simulink model "Modulator_Xilinx_Verilog"  (Simulink 7.8)
settings: Solver=VariableStepDiscrete  StartTime=0.0  StopTime=100/25000000  RelTol=1e-3
undefined symbols (not defined in the file): gcbh, xlBlockLoadCallback, xlipgetpartsetting
libraries: xbsIndex_r4 x11
settings Model: Creator=Cedric  LastModifiedBy=Cedric

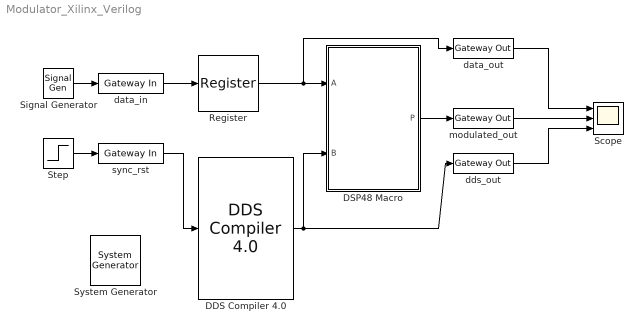
== system Modulator_Xilinx_Verilog ==
  " System Generator" : xbsIndex_r4/ System Generator  Tag=genX  xilinxfamily=virtex6  part=xc6vlx240t  speed=-1  package=ff1156  synthesis_tool=XST  clock_wrapper=Clock Enables  directory=./netlist  proj_type=Project Navigator  Synth_file=XST Defaults  Impl_file=ISE Defaults  testbench=off  simulink_period=1/25000000  sysclk_period=10  dcm_input_clock_period=10  incr_netlist=off  trim_vbits=Everywhere in SubSystem  dbl_ovrd=According to Block Masks  core_generation=According to Block Masks  run_coregen=off  deprecated_control=off  eval_field=0  block_type=sysgen
  "DDS Compiler 4.0 " : xbsIndex_r4/DDS Compiler 4.0   partspresent=Phase_Generator_and_SIN_COS_LUT  dds_clock_rate=100  channels=1  parameter_entry=System_Parameters  spurious_free_dynamic_range=36  frequency_resolution=0.4  noise_shaping=None  phase_width=28  output_width=6  output_selection=Sine  negative_sine=off  negative_cosine=off  amplitude_mode=Full_Range  memory_type=Block_ROM  optimization_goal=Auto  dsp48_use=Maximal  latency_configuration=Auto  latency=2  has_phase_out=off  sclr_pin=on  clock_enable=off  rfd=off  rdy=off  channel_pin=off  explicit_period=off  period=1  phase_increment=Fixed  output_frequency1=5  output_frequency2=0  output_frequency3=0  output_frequency4=0  output_frequency5=0  output_frequency6=0  output_frequency7=0  output_frequency8=0  output_frequency9=0  output_frequency10=0  output_frequency11=0  output_frequency12=0  output_frequency13=0  output_frequency14=0  output_frequency15=0  output_frequency16=0  pinc1='0'  pinc2='0'  pinc3='0'  pinc4='0'  pinc5='0'  pinc6='0'  pinc7='0'  pinc8='0'  pinc9='0'  pinc10='0'  pinc11='0'  pinc12='0'  pinc13='0'  pinc14='0'  pinc15='0'  pinc16='0'  phase_offset=None  phase_offset_angles1=0  phase_offset_angles2=0  phase_offset_angles3=0  phase_offset_angles4=0  phase_offset_angles5=0  phase_offset_angles6=0  phase_offset_angles7=0  phase_offset_angles8=0  phase_offset_angles9=0  phase_offset_angles10=0  phase_offset_angles11=0  phase_offset_angles12=0  phase_offset_angles13=0  phase_offset_angles14=0  phase_offset_angles15=0  phase_offset_angles16=0  poff1='0'  poff2='0'  poff3='0'  poff4='0'  poff5='0'  poff6='0'  poff7='0'  poff8='0'  poff9='0'  poff10='0'  poff11='0'  poff12='0'  poff13='0'  poff14='0'  poff15='0'  poff16='0'  por_mode=false  gui_behaviour=Sysgen  ip_name=DDS Compiler  ip_version=4.0  dsptool_ready=true  wrapper_available=true  port_translation_map={ 'ce' => 'en', 'sclr' => 'rst' }  ipcore_xco_need_fpga_part=true  ipcore_fpga_part=xlipgetpartsetting(gcb, {'virtex4', 'xc4vsx35', '-10', 'ff668'})  ipcore_usecache=true  ipcore_useipmodelcache=true  ipcore_verbose=false  block_type=dds_compiler_v4_0
  DSP48 Macro : Subsystem  LoadFcn=xlBlockLoadCallback(gcbh);  mask(Xilinx DSP48 Macro Block){infoedit=Macro function to simplify use of the DSP48 primitive, especially as a dynamic operator, portalist=A, portblist=B, portclist=No, instrlist=|, pipeline_sgadvanced=, pipeline=Custom, pipeachoices_sgadvanced=, pipeachoices=1, pipebchoices_sgadvanced=, pipebchoices=1, pipecchoices_sgadvanced=, pipecchoices=on, pipepchoices_sgadvanced=, pipepchoices=on, pipemchoices_sgadvanced=, pipemchoices=on, pipectrlchoices_sgadvanced=, pipectrlchoices=on, pipemuxachoices_sgadvanced=, pipemuxachoices=0, pipemuxbchoices_sgadvanced=, pipemuxbchoices=0, pipemuxcchoices_sgadvanced=, pipemuxcchoices=0, pipemuxctrlchoices_sgadvanced=, pipemuxctrlchoices=0, pipeline_array_flag_sgadvanced=, pipeline_array_flag=off, custom_pipeline_cache=[1  1  1  1  1  1  0  0  0  0], precision_sgadvanced=, precision=Full, arith_type_sgadvanced=, arith_type=Unsigned, n_bits=8, bin_pt=2, bcout_sgadvanced=, bcout=off, acout_sgadvanced=, acout=off, carryout_sgadvanced=, carryout=off, carrycascout_sgadvanced=, carrycascout=off, pcout_sgadvanced=, pcout=off, rst_all_sgadvanced=, rst_all=off, rst_a_sgadvanced=, rst_a=off, rst_b_sgadvanced=, rst_b=off, rst_c_sgadvanced=, rst_c=off, rst_m_sgadvanced=, rst_m=off, rst_p_sgadvanced=, rst_p=off, rst_ctrl_sgadvanced=, rst_ctrl=off, ce_all_sgadvanced=, ce_all=off, ce_a_sgadvanced=, ce_a=off, ce_b_sgadvanced=, ce_b=off, ce_c_sgadvanced=, ce_c=off, ce_m_sgadvanced=, ce_m=off, ce_p_sgadvanced=, ce_p=off, ce_ctrl_sgadvanced=, ce_ctrl=off, dbl_ovrd_sgadvanced=, dbl_ovrd=off, synth_opt_sgadvanced=, synth_opt=on, errorlist=false, statestr=8748f9e4e14b4b54c46918fee19c673c, explicit_period=, period=1, maskdoc=, has_advanced_control=0, sggui_pos=-1,-1,-1,-1, block_type=dsp48macro, block_version=8.2.1, sg_icon_stat=90,142,2,1,white,blue,0,7afd0e130bd830a51d6376b21eaeb333,right,,[ ],[ ], sg_mask_display=|, sg_list_contents=, sg_blockgui_xml=}
      mask instrlist=|
      | <!DOCTYPE HTML PUBLIC "-//W3C//DTD HTML 4.0//EN" "http://www.w3.org/TR/REC-html40/strict.dtd">
      | <html><head><meta name="qrichtext" content="1" /><style type="text/css">
      | p, li { white-space: pre-wrap; }
      | </style></head><body style=" font-family:'MS Shell Dlg 2'; font-size:8.25pt; font-weight:400; font-style:normal;">
      | <p style=" margin-top:12px; margin-bottom:12px; margin-left:0px; margin-right:0px; -qt-block-indent:0; text-indent:0px;"><span style=" font-family:'MS Shell Dlg'; font-size:8pt;">P=A*B</span></p></body></html>
      mask sg_mask_display=|
      | fprintf('','COMMENT: begin icon graphics');
      | patch([0 90 90 0 0 ],[0 0 142 142 0 ],[0.77 0.82 0.91 ]);
      | plot([0 90 90 0 0 ],[0 0 142 142 0 ]);
      | patch([18.3 35.64 47.64 59.64 71.64 47.64 30.3 18.3 ],[84.32 84.32 96.32 84.32 96.32 96.32 96.32 84.32 ],[1 1 1 ]);
      | patch([30.3 47.64 35.64 18.3 30.3 ],[72.32 72.32 84.32 84.32 72.32 ],[0.931 0.946 0.973 ]);
      | patch([18.3 35.64 47.64 30.3 18.3 ],[60.32 60.32 72.32 72.32 60.32 ],[1 1 1 ]);
      | patch([30.3 71.64 59.64 47.64 35.64 18.3 30.3 ],[48.32 48.32 60.32 48.32 60.32 60.32 48.32 ],[0.931 0.946 0.973 ]);
      | fprintf('','COMMENT: end icon graphics');
      | fprintf('','COMMENT: begin icon text');
      | color('black');port_label('input',1,'A');
      | color('black');port_label('input',2,'B');
      | color('black');port_label('output',1,'P');
      | fprintf('','COMMENT: end icon text');
      mask prompts: infoedit ""; portalist "Inputs to port <tt>A</tt>"; portblist "Inputs to port <tt>B</tt>"; portclist "Inputs to port <tt>C</tt>"; instrlist "Instructions"; pipeline_sgadvanced ""; pipeline "Pipeline options"; pipeachoices_sgadvanced ""; pipeachoices "<tt>A</tt>"; pipebchoices_sgadvanced ""; pipebchoices "<tt>B</tt>"; pipecchoices_sgadvanced ""; pipecchoices "<tt>C</tt>"; pipepchoices_sgadvanced ""; pipepchoices "<tt>P</tt>"; pipemchoices_sgadvanced ""; pipemchoices "Multiplier"; pipectrlchoices_sgadvanced ""; pipectrlchoices "Controls (<tt>opmode</tt>, <tt>subtract</tt>,<br> <tt>carry_in</tt>, <tt>carry_in_sel</tt>)"; pipemuxachoices_sgadvanced ""; pipemuxachoices "MuxA"; pipemuxbchoices_sgadvanced ""; pipemuxbchoices "MuxB"; pipemuxcchoices_sgadvanced ""; pipemuxcchoices "MuxC"; pipemuxctrlchoices_sgadvanced ""; pipemuxctrlchoices "MuxCtrl"; pipeline_array_flag_sgadvanced ""; pipeline_array_flag "Define Using Array"; custom_pipeline_cache "Custom Pipeline Options([A,B,C,P,Ctrl,M,MuxA,MuxB,MuxC,MuxCtrl])"; precision_sgadvanced ""; arith_type_sgadvanced ""; arith_type "Output type"; n_bits "Number of bits"; bin_pt "Binary point"; bcout_sgadvanced ""; bcout "<tt>BCOUT</tt>"; acout_sgadvanced ""; acout "<tt>ACOUT</tt>"; carryout_sgadvanced ""; carryout "<tt>CARRYOUT</tt>"; carrycascout_sgadvanced ""; carrycascout "<tt>CARRYCASCOUT</tt>"; pcout_sgadvanced ""; pcout "<tt>PCOUT</tt>"; rst_all_sgadvanced ""; rst_all "<tt>Global Reset</tt>"; rst_a_sgadvanced ""; rst_a "Reset port for <tt>A</tt>"; rst_b_sgadvanced ""; rst_b "Reset port for <tt>B</tt>"; rst_c_sgadvanced ""; rst_c "Reset port for <tt>C</tt>"; rst_m_sgadvanced ""; rst_m "Reset port for multiplier"; rst_p_sgadvanced ""; rst_p "Reset port for <tt>P</tt>"; rst_ctrl_sgadvanced ""; rst_ctrl "Reset port for controls <br> (<tt>opmode</tt>, <tt>subtract</tt>,<br> <tt>carry_in</tt>, <tt>carry_in_sel</tt>)"; ce_all_sgadvanced ""; ce_all "<tt>Global Enable</tt>"; ce_a_sgadvanced ""; ce_a "Enable port for <tt>A</tt>"; ce_b_sgadvanced ""; ce_b "Enable port for <tt>B</tt>"; ce_c_sgadvanced ""; ce_c "Enable port for <tt>C</tt>"; ce_m_sgadvanced ""; ce_m "Enable port for multiplier"; ce_p_sgadvanced ""; ce_p "Enable port for <tt>P</tt>"; ce_ctrl_sgadvanced ""; ce_ctrl "Enable port for controls <br> (<tt>opmode</tt>, <tt>subtract</tt>,<br> <tt>carry_in</tt>, <tt>carry_in_sel</tt>)"; dbl_ovrd_sgadvanced ""; dbl_ovrd "Override with doubles"; synth_opt_sgadvanced ""; synth_opt "Use DSP48"; errorlist ""; statestr ""; explicit_period ""; period ""; maskdoc ""; has_advanced_control ""; sggui_pos ""; block_type ""; block_version ""; sg_icon_stat ""; sg_mask_display ""; sg_list_contents ""; sg_blockgui_xml ""
      mask help: Macro function to simplify use of the DSP48 primitive, especially as a dynamic operator
      mask init:
      | try
      |   tmp_gcb = gcb;
      |   tmp_gcbh = gcbh;
      |   if (strcmp('SysGenIndex',get_param(bdroot(tmp_gcbh),'tag')) && ~isempty(regexp(bdroot(tmp_gcb), '^xbs', 'once')))
      |     return;
      |   end;
      |   xlMungeMaskParams;
      | 
      |   block_type='dsp48macro';
      | 
      |   serialized_declarations = '{''block_type''=>''String''}';
      |   xldsp48macro_init();
      |   ptable_ = xlblockprep(get_param(tmp_gcb, 'MaskWSVariables'));
      |   try
      |     xlBlockMoveCallback(tmp_gcbh);
      |   catch 
      |      clear global xl_updateicon_recursion_guard;
      |   end;
      | catch
      |   global dbgsysgen;
      |   if(~isempty(dbgsysgen) && dbgsysgen)
      |     e = regexprep(lasterr, '\n', '\nError: ');
      |     disp(['Error: While running MaskInit code on block ' tmp_gcb ': ' e]);
      |     error(e);
      |   end
      | end
      settings: CopyFcn=tmp_gcbh = gcbh;set_param(tmp_gcbh,'linkstatus','none');xlBlockMoveCallback(gcbh);  DeleteFcn=xlDestroyGui(gcbh);  ModelCloseFcn=xlDestroyGui(gcbh);  PreSaveFcn=xlBlockPreSaveCallback(gcbh);  PostSaveFcn=xlBlockPostSaveCallback(gcbh);  DestroyFcn=xlDestroyGui(gcbh);  OpenFcn=xlOpenGui(gcbh, 'dsp48macro_gui.xml', @dsp48macroenablement, @dsp48macroaction)  CloseFcn=xlDestroyGui(gcbh);  MoveFcn=xlBlockMoveCallback(gcbh);
      mask Help: eval('');xlDoc('-book','sysgen','-topic','DSP48_Macro');
      mask StyleString: edit,edit,edit,edit,edit,edit,popup(External Registers|No External Registers|Custom),edit,popup(0|1|2),edit,popup(0|1|2),edit,checkbox,edit,checkbox,edit,checkbox,edit,checkbox,edit,popup(0|1|2),edit,popup(0|1|2),edit,popup(0|1|2),edit,popup(0|1|2),edit,checkbox,edit,edit,popup(Full|User Defined),edit,popup(Signed  (2's comp)|Unsigned),edit,edit,edit,checkbox,edit,checkbox,edit,checkbox,edit,checkbox,edit,checkbox,edit,checkbox,edit,checkbox,edit,checkbox,edit,checkbox,edit,checkbox,edit,checkbox,edit,checkbox,edit,checkbox,edit,checkbox,edit,checkbox,edit,checkbox,edit,checkbox,edit,checkbox,edit,checkbox,edit,checkbox,edit,checkbox,edit,edit,edit,edit,edit,edit,edit,edit,edit,edit,edit,edit,edit
      mask Display:
      | fprintf('','COMMENT: begin icon graphics');
      | patch([0 90 90 0 0 ],[0 0 142 142 0 ],[0.77 0.82 0.91 ]);
      | plot([0 90 90 0 0 ],[0 0 142 142 0 ]);
      | patch([18.3 35.64 47.64 59.64 71.64 47.64 30.3 18.3 ],[84.32 84.32 96.32 84.32 96.32 96.32 96.32 84.32 ],[1 1 1 ]);
      | patch([30.3 47.64 35.64 18.3 30.3 ],[72.32 72.32 84.32 84.32 72.32 ],[0.931 0.946 0.973 ]);
      | patch([18.3 35.64 47.64 30.3 18.3 ],[60.32 60.32 72.32 72.32 60.32 ],[1 1 1 ]);
      | patch([30.3 71.64 59.64 47.64 35.64 18.3 30.3 ],[48.32 48.32 60.32 48.32 60.32 60.32 48.32 ],[0.931 0.946 0.973 ]);
      | fprintf('','COMMENT: end icon graphics');
      | fprintf('','COMMENT: begin icon text');
      | color('black');port_label('input',1,'A');
      | color('black');port_label('input',2,'B');
      | color('black');port_label('output',1,'P');
      | fprintf('','COMMENT: end icon text');
  Register : xbsIndex_r4/Register  init=0  rst=off  en=off  dbl_ovrd=off  block_type=register
  Scope : Scope  NumInputPorts=3
      settings: YMin=-5~-5~-5  YMax=5~5~5
  Signal Generator : SignalGenerator  WaveForm=square  Frequency=500000
  Step : Step  Time=1/25000000  Before=1  After=0  SampleTime=1/25000000
  data_in : xbsIndex_r4/Gateway In  gui_display_data_type=Fixed-point  arith_type="Signed  (2's comp)"  n_bits=16  bin_pt=14  preci_type=Single  exp_width=8  frac_width=24  quantization="Round  (unbiased: +/- Inf)"  overflow=Saturate  period=1/25000000  dbl_ovrd=off  timing_constraint=None  locs_specified=off  LOCs={}  UseAsADC=off  ADCChannel='1'  inherit_from_input=off  hdl_port=on  block_type=gatewayin
  data_out : xbsIndex_r4/Gateway Out  inherit_from_input=off  hdl_port=on  timing_constraint=None  locs_specified=off  LOCs={}  UseAsDAC=off  DACChannel='1'  block_type=gatewayout
  dds_out : xbsIndex_r4/Gateway Out  inherit_from_input=off  hdl_port=on  timing_constraint=None  locs_specified=off  LOCs={}  UseAsDAC=off  DACChannel='1'  block_type=gatewayout
  modulated_out : xbsIndex_r4/Gateway Out  inherit_from_input=off  hdl_port=on  timing_constraint=None  locs_specified=off  LOCs={}  UseAsDAC=off  DACChannel='1'  block_type=gatewayout
  sync_rst : xbsIndex_r4/Gateway In  gui_display_data_type=Boolean  arith_type=Boolean  n_bits=16  bin_pt=14  preci_type=Single  exp_width=8  frac_width=24  quantization="Round  (unbiased: +/- Inf)"  overflow=Saturate  period=1/25000000  dbl_ovrd=off  timing_constraint=None  locs_specified=off  LOCs={}  UseAsADC=off  ADCChannel='1'  inherit_from_input=off  hdl_port=on  block_type=gatewayin
  wires:
  data_in/1 -> Register/1
  Signal Generator/1 -> data_in/1
  Register/1 -> DSP48 Macro/1(A), data_out/1
  data_out/1 -> Scope/1
  DSP48 Macro/1(P) -> modulated_out/1
  modulated_out/1 -> Scope/2
  dds_out/1 -> Scope/3
  sync_rst/1 -> "DDS Compiler 4.0 "/1
  "DDS Compiler 4.0 "/1 -> DSP48 Macro/2(B), dds_out/1
  Step/1 -> sync_rst/1

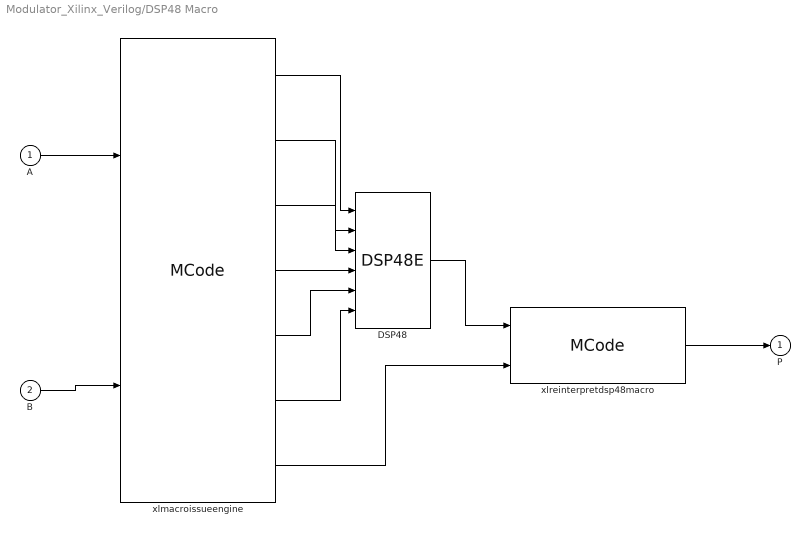
== system Modulator_Xilinx_Verilog/DSP48 Macro ==
  A : Inport
  B : Inport  Port=2
  DSP48 : xbsIndex_r4/DSP48E  use_a=Direct from A Port  use_b=Direct from B Port  reset_preg=off  pattern_from_creg=on  pattern='000000000000'  mask_from_creg=on  pattern_mask='000000000000'  sel_rounding_mask=Select mask  use_op=off  use_creg=off  rst_all=off  en_all=off  use_pcin=off  use_carrycascin=off  use_multsignin=off  use_carryout=off  use_patterndetect=off  use_patternbdetect=off  use_overflow=off  use_underflow=off  use_acout=off  use_bcout=off  use_pcout=off  use_multsignout=off  use_carrycascout=off  pipeline_a=1  pipeline_b=1  pipeline_acout=1  pipeline_bcout=1  pipeline_c=off  pipeline_p=on  pipeline_mult=on  pipeline_opmode=on  pipeline_alumode=on  pipeline_carryin=on  pipeline_carryinsel=on  rst_a=off  rst_b=off  rst_c=off  rst_mult=off  rst_p=off  rst_carry_in=off  rst_alumode=off  rst_ctrl=off  en_a1=off  en_a2=off  en_b1=off  en_b2=off  en_c=off  en_mult=off  en_p=off  en_carry_in=off  en_alumode=off  en_multcarryin=off  en_ctrl=off  use_synth_model=off  addsub_mode=ONE48  xl_useadderonly=off  block_type=dsp48e
  xlmacroissueengine : xbsIndex_r4/MCode  mfname=xlissue_engine_v5  explicit_period=off  period=inf  dbl_ovrd=off  enable_stdout=off  enable_debug=off  suppress_output=on  defparams={'id_a1', 0,'id_a2', 0,'id_a3', 0,'id_a4', 0,'id_a5', 0,'id_a6', 0,'id_a7', 0,'id_b1', 0,'id_b2', 0,'id_b3', 0,'id_b4', 0,'id_b5', 0,'id_b6', 0,'id_b7', 0,'id_c0', 0,'id_c1', 0,'id_c2', 0,'id_c3', 0,'id_c4', 0,'id_c5', 0,'id_c6', 0,'id_c7', 0,'op_const0',5,'op_const1', 0,'op_const2', 0,'op_const3', 0,'op_const4', 0,'op_const5', 0,'op_const6', 0,'op_const7', 0,'alumode_const0',0,'alumode_const1', 0,'alumode_const2', 0,'alumode_const3', 0,'alumode_const4', 0,'alumode_const5', 0,'alumode_const6', 0,'alumode_const7', 0,'carry_in_sel0',0,'carry_in_sel1', 0,'carry_in_sel2', 0,'carry_in_sel3', 0,'carry_in_sel4', 0,'carry_in_sel5', 0,'carry_in_sel6', 0,'carry_in_sel7', 0,'external_cin0', 0,'external_cin1', 0,'external_cin2', 0,'external_cin3', 0,'external_cin4', 0,'external_cin5', 0,'external_cin6', 0,'external_cin7', 0,'reg_a',0,'reg_b',0,'reg_c',0,'reg_op',0,'mode0', 1,'mode1', 0,'mode2', 0,'mode3', 0,'mode4', 0,'mode5', 0,'mode6', 0,'mode7', 0,'ce_all',true,'use_ce_all',false,'sel',0,'rst_all',false,'use_rst_all',false,'cinused',false,'ninstr',1}  hide_port_list={'c'}  block_type=mcode
      settings: xl_area=[0, 0, 0, 0, 0, 0, 0]
  xlreinterpretdsp48macro : xbsIndex_r4/MCode  mfname=xlreinterpretdsp48macro  explicit_period=off  period=1  dbl_ovrd=off  enable_stdout=off  enable_debug=off  suppress_output=off  defparams={'full',precision,'n_bits',n_bits,'bin_pt',bin_pt,'arith_type',arith_type}  hide_port_list={}  block_type=mcode
      settings: xl_area=[0, 0, 0, 0, 0, 0, 0]
  P : Outport
  wires:
  xlreinterpretdsp48macro/1 -> P/1
  DSP48/1 -> xlreinterpretdsp48macro/1
  xlmacroissueengine/7 -> xlreinterpretdsp48macro/2
  xlmacroissueengine/6 -> DSP48/6
  xlmacroissueengine/5 -> DSP48/5
  xlmacroissueengine/4 -> DSP48/4
  xlmacroissueengine/3 -> DSP48/3
  xlmacroissueengine/2 -> DSP48/2
  xlmacroissueengine/1 -> DSP48/1
  B/1 -> xlmacroissueengine/2
  A/1 -> xlmacroissueengine/1
